simulink model "sim_variable_structure2"  (R2020a)
settings: Solver=FixedStepAuto  StartTime=0.0  StopTime=end_time  FixedStep=FStep  RelTol=1e-3
undefined symbols (not defined in the file): b, c, T1, T2, T3
libraries: simulink_extras x3
settings Model: Creator=ogure  LastModifiedBy=my000
settings SolverCC: SolverResetMethod=Robust
settings DataIOCC: SaveFormat=Array  SaveOutput=off  SignalLogging=off  ReturnWorkspaceOutputs=off
settings DebuggingCC: SolverPrmCheckMsg=warning
settings SFSimCC: CustomCodeUndefinedFunction=UseInterfaceOnly

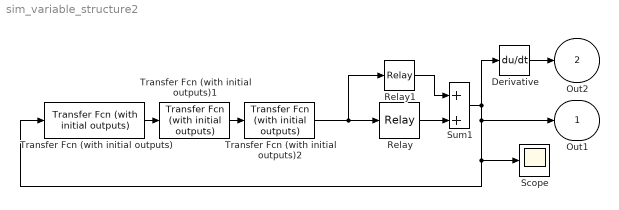
== system sim_variable_structure2 ==
  Derivative : Derivative
  Relay : Relay  OnSwitchValue=b  OffSwitchValue=b  OnOutputValue=c
  Relay1 : Relay  OnSwitchValue=-b  OffSwitchValue=-b  OnOutputValue=0  OffOutputValue=-c
  Scope : Scope
  Sum1 : Sum  Inputs=|++
  Transfer Fcn (with initial outputs) : simulink_extras/Additional Linear/Transfer Fcn (with initial outputs)  N=[1]  D="[T1  1]"  Y0=0  U0=100
  Transfer Fcn (with initial outputs)1 : simulink_extras/Additional Linear/Transfer Fcn (with initial outputs)  N=[1]  D="[T2  1]"  Y0=0  U0=0
  Transfer Fcn (with initial outputs)2 : simulink_extras/Additional Linear/Transfer Fcn (with initial outputs)  N=[1]  D="[T3  1]"  Y0=0  U0=0
  Out1 : Outport  SignalName=x  VectorParamsAs1DForOutWhenUnconnected=off
  Out2 : Outport  Port=2  SignalName=y  VectorParamsAs1DForOutWhenUnconnected=off
  wires:
  Derivative/1 -> Out2/1
  Relay/1 -> Sum1/2
  Sum1/1 -> Transfer Fcn (with initial outputs)/1, Scope/1, Out1/1, Derivative/1
  Transfer Fcn (with initial outputs)/1 -> Transfer Fcn (with initial outputs)1/1
  Transfer Fcn (with initial outputs)1/1 -> Transfer Fcn (with initial outputs)2/1
  Relay1/1 -> Sum1/1
  Transfer Fcn (with initial outputs)2/1 -> Relay1/1, Relay/1
